simulink model "MPC_IL"  (R2018a)
settings: Solver=VariableStepAuto  StartTime=0.0  StopTime=100  FixedStep=.025  RelTol=1e-3
InitFcn:
  | param
undefined symbols (not defined in the file or in its folder): animation, control, P
libraries: simulink x2
settings Model: Creator=Mat Haskell  LastModifiedBy=mat
settings CodeAppCC: StateflowObjectComments=on

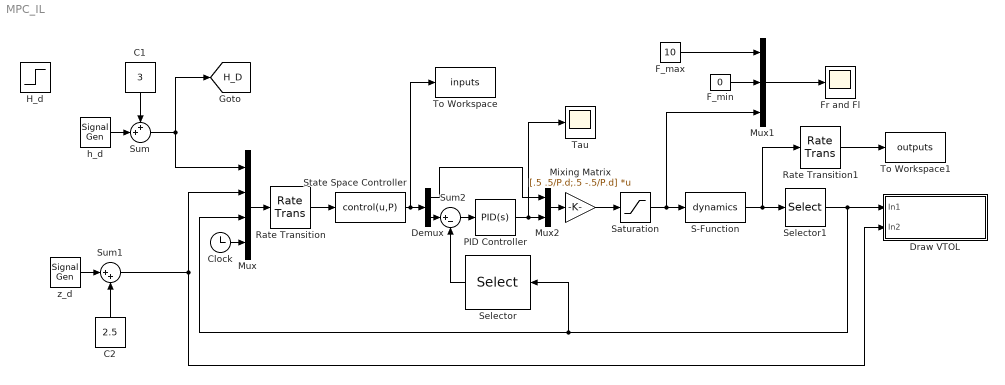
== system MPC_IL ==
  C1 : Constant  Value=3
  C2 : Constant  Value=2.5
  Clock : Clock
  Demux : Demux  Outputs=2
  Draw VTOL : Subsystem
  F_max : Constant  Value=10
  F_min : Constant  Value=0
  Fr and Fl : Scope
  H_d : Step  Time=0  After=0  SampleTime=0
  Mixing Matrix : Gain  Gain=[.5 .5/P.d;.5 -.5/P.d]  Multiplication=Matrix(K*u)
  Mux : Mux
  Mux1 : Mux  Inputs=3
  Mux2 : Mux  Inputs=2
  PID Controller : simulink/Continuous/PID Controller  Controller=PID  TimeDomain=Continuous-time  SampleTime=-1  IntegratorMethod=Forward Euler  FilterMethod=Forward Euler  Form=Parallel  UseFilter=on  ControllerParametersSource=internal  P=P.kptheta  I=0  D=P.kdtheta  N=100  InitialConditionSource=internal  InitialConditionForIntegrator=0  InitialConditionForFilter=0  ExternalReset=none  LimitOutput=off  UpperSaturationLimit=inf  LowerSaturationLimit=-inf  LinearizeAsGain=on  AntiWindupMode=none  Kb=1  TrackingMode=off  Kt=1  PParamMin=[]  PParamMax=[]  IParamMin=[]  IParamMax=[]  DParamMin=[]  DParamMax=[]  NParamMin=[]  NParamMax=[]  KbParamMin=[]  KbParamMax=[]  KtParamMin=[]  KtParamMax=[]  POutMin=[]  POutMax=[]  IOutMin=[]  IOutMax=[]  DOutMin=[]  DOutMax=[]  NOutMin=[]  NOutMax=[]  KbOutMin=[]  KbOutMax=[]  KtOutMin=[]  KtOutMax=[]  IntegratorOutMin=[]  IntegratorOutMax=[]  FilterOutMin=[]  FilterOutMax=[]  SumOutMin=[]  SumOutMax=[]  SumI1OutMin=[]  SumI1OutMax=[]  SumI2OutMin=[]  SumI2OutMax=[]  SumI3OutMin=[]  SumI3OutMax=[]  SumDOutMin=[]  SumDOutMax=[]  SaturationOutMin=[]  SaturationOutMax=[]  IntegratorContinuousStateAttributes=''  IntegratorStateMustResolveToSignalObject=off  IntegratorRTWStateStorageClass=Auto  FilterContinuousStateAttributes=''  FilterStateMustResolveToSignalObject=off  FilterRTWStateStorageClass=Auto  DifferentiatorICPrevScaledInput=0  DifferentiatorOutMin=[]  DifferentiatorOutMax=[]  FilterDiffOutCoefMin=[]  FilterDiffOutCoefMax=[]  SumDenOutMin=[]  SumDenOutMax=[]  SumNumOutMin=[]  SumNumOutMax=[]  ReciprocalOutMin=[]  ReciprocalOutMax=[]  DivideOutMin=[]  DivideOutMax=[]  TunerSelectOption=Transfer Function Based (PID Tuner App)
  Rate Transition : RateTransition  OutPortSampleTime=P.ts
  Rate Transition1 : RateTransition  OutPortSampleTime=P.ts
  S-Function : S-Function  FunctionName=dynamics  Parameters=P  SFunctionDeploymentMode=off  EnableBusSupport=off
  Saturation : Saturate  UpperLimit=10  LowerLimit=0
  Selector : Selector  InputPortWidth=6  IndexOptions=Index vector (dialog)  Indices=[3]  OutputSizes=1
  Selector1 : Selector  InputPortWidth=9  IndexOptions=Index vector (dialog)  Indices=[1 2 3 4 5 6]  OutputSizes=1
  State Space Controller : MATLABFcn  MATLABFcn=control(u,P)
  Sum : Sum  Inputs=++|
  Sum1 : Sum  Inputs=|++
  Sum2 : Sum  Inputs=|+-
  Tau : Scope
  To Workspace : ToWorkspace  VariableName=inputs  SaveFormat=Structure With Time  SampleTime=-1
  To Workspace1 : ToWorkspace  VariableName=outputs  SaveFormat=Structure With Time  SampleTime=-1
  h_d : SignalGenerator  WaveForm=square  Amplitude=2  Frequency=.05
  z_d : SignalGenerator  WaveForm=square  Amplitude=2.5  Frequency=.04
  tag scope: H_D=global
  wires:
  C1/1 -> Sum/1
  Sum/1 -> Mux/1, [H_D]
  z_d/1 -> Sum1/1
  C2/1 -> Sum1/2
  Sum1/1 -> Mux/2, Draw VTOL/2(In2)
  Mux1/1 -> Fr and Fl/1
  F_min/1 -> Mux1/2
  F_max/1 -> Mux1/1
  Saturation/1 -> Mux1/3, S-Function/1
  h_d/1 -> Sum/2
  S-Function/1 -> Selector1/1, Rate Transition1/1
  Clock/1 -> Mux/4
  Mixing Matrix/1 -> Saturation/1
  State Space Controller/1 -> To Workspace/1, Demux/1
  Demux/1 -> Mux2/1
  Mux2/1 -> Mixing Matrix/1
  PID Controller/1 -> Tau/1, Mux2/2
  Mux/1 -> Rate Transition/1
  Rate Transition/1 -> State Space Controller/1
  Demux/2 -> Sum2/1
  Sum2/1 -> PID Controller/1
  Selector/1 -> Sum2/2
  Rate Transition1/1 -> To Workspace1/1
  Selector1/1 -> Draw VTOL/1(In1), Selector/1, Mux/3

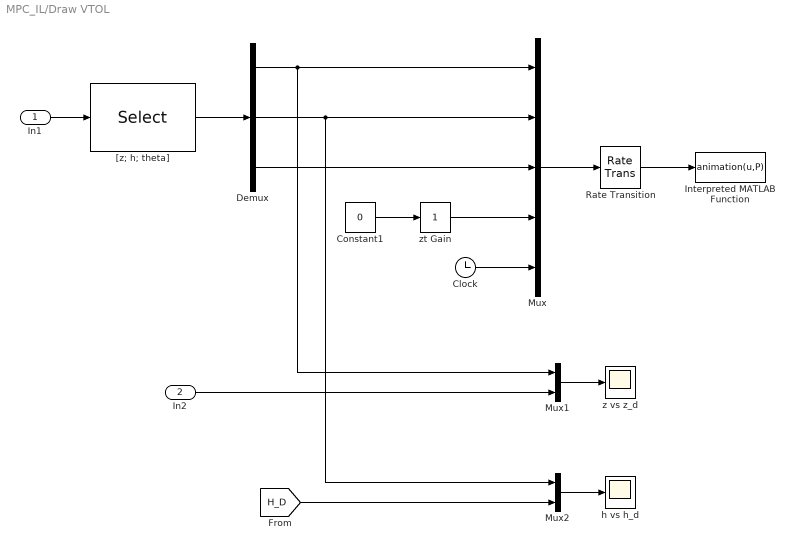
== system MPC_IL/Draw VTOL ==
  In1 : Inport
  In2 : Inport  Port=2
  Clock : Clock
  Constant1 : Constant  Value=0
  Demux : Demux  Outputs=3
  Interpreted MATLAB Function : MATLABFcn  MATLABFcn=animation(u,P)  OutputDimensions=0
  Mux : Mux  Inputs=5
  Mux1 : Mux  Inputs=2
  Mux2 : Mux  Inputs=2
  Rate Transition : RateTransition  OutPortSampleTime=P.t_plot
  "[z; h; theta]" : Selector  InputPortWidth=6  IndexOptions=Index vector (dialog)  Indices=[1 2 3]  OutputSizes=1
  h vs h_d : Scope
  z vs z_d : Scope
  zt Gain : simulink/Math Operations/Slider Gain  gain=1  low=0  high=5
  wires:
  Demux/1 -> Mux1/1, Mux/1
  Demux/2 -> Mux2/1, Mux/2
  Demux/3 -> Mux/3
  Rate Transition/1 -> Interpreted MATLAB Function/1
  Mux/1 -> Rate Transition/1
  zt Gain/1 -> Mux/4
  Constant1/1 -> zt Gain/1
  Clock/1 -> Mux/5
  In2/1 -> Mux1/2
  Mux1/1 -> z vs z_d/1
  Mux2/1 -> h vs h_d/1
  [H_D] -> Mux2/2
  In1/1 -> "[z; h; theta]"/1
  "[z; h; theta]"/1 -> Demux/1
